simulink model "final_model_test"  (R2015a)
settings: Solver=ode3  StartTime=0.0  StopTime=10  RelTol=1e-3
settings Model: Creator=BML  LastModifiedBy=BML
settings SolverCC: AutoInsertRateTranBlk=on
settings DebuggingCC: AlgebraicLoopMsg=error  ArtificialAlgebraicLoopMsg=none  MaxConsecutiveZCsMsg=none
settings ModelReferenceCC: ModelReferenceMinAlgLoopOccurrences=on

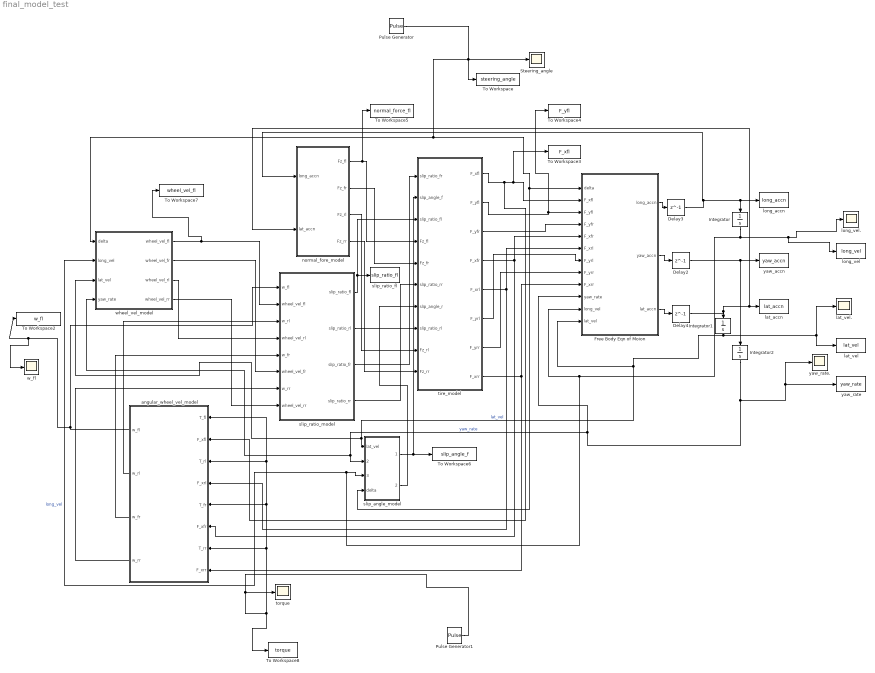
== system final_model_test ==
  "           Steering_angle" : Scope
      settings: SaveName=ScopeData8
  "           torque" : Scope
      settings: SaveName=ScopeData10
  Delay2 : Delay  DelayLength=1  SampleTime=1
  Delay3 : Delay  DelayLength=1  SampleTime=1
  Delay4 : Delay  DelayLength=1  SampleTime=1
  Free Body Eqn of Moion : Subsystem
  Integrator : Integrator  InitialCondition=22.22
  Integrator1 : Integrator
  Integrator2 : Integrator
  Pulse Generator : DiscretePulseGenerator  PulseType=Time based  Amplitude=0  Period=8  PulseWidth=5  PhaseDelay=3
  Pulse Generator1 : DiscretePulseGenerator  Amplitude=50  Period=8  PulseWidth=5  PhaseDelay=3
  To Workspace : ToWorkspace  VariableName=steering_angle  SaveFormat=Timeseries  SampleTime=1
  To Workspace2 : ToWorkspace  VariableName=w_fl  SaveFormat=Timeseries  SampleTime=1
  To Workspace3 : ToWorkspace  VariableName=F_xfl  SaveFormat=Timeseries  SampleTime=1
  To Workspace4 : ToWorkspace  VariableName=F_yfl  SaveFormat=Timeseries  SampleTime=1
  To Workspace5 : ToWorkspace  VariableName=normal_force_fl  SaveFormat=Timeseries  SampleTime=1
  To Workspace6 : ToWorkspace  VariableName=slip_angle_f  SaveFormat=Timeseries  SampleTime=1
  To Workspace7 : ToWorkspace  VariableName=wheel_vel_fl  SaveFormat=Timeseries  SampleTime=1
  To Workspace8 : ToWorkspace  VariableName=torque  SaveFormat=Timeseries  SampleTime=-1
  angular_wheel_vel_model : Subsystem
  lat_accn : ToWorkspace  VariableName=lat_accn  SaveFormat=Timeseries  SampleTime=1
  lat_vel : ToWorkspace  VariableName=lat_vel  SaveFormat=Timeseries  SampleTime=1
  lat_vel. : Scope
  long_accn : ToWorkspace  VariableName=long_accn  SaveFormat=Timeseries  SampleTime=1
  long_vel : ToWorkspace  VariableName=long_vel  SaveFormat=Timeseries  SampleTime=1
  long_vel. : Scope
  normal_fore_model : Subsystem
  slip_angle_model : Subsystem
  slip_ratio_fl : ToWorkspace  VariableName=slip_ratio_fl  SaveFormat=Timeseries  SampleTime=1
  slip_ratio_model : Subsystem
  tire_model : Subsystem
  w_fl : Scope
      settings: SaveName=ScopeData5
  wheel_vel_model : Subsystem
  yaw_accn : ToWorkspace  VariableName=yaw_accn  SaveFormat=Timeseries  SampleTime=1
  yaw_rate : ToWorkspace  VariableName=yaw_rate  SaveFormat=Timeseries  SampleTime=1
  yaw_rate. : Scope
      settings: SaveName=ScopeData2
  wires:
  slip_ratio_model/1(slip_ratio_fl) -> slip_ratio_fl/1, tire_model/3(slip_ratio_fl)
  slip_ratio_model/2(slip_ratio_rl) -> tire_model/8(slip_ratio_rl)
  Integrator2/1 -> Free Body Eqn of Moion/10(yaw_rate), slip_angle_model/2(yaw_rate), wheel_vel_model/4(yaw_rate), yaw_rate./1, yaw_rate/1  "yaw_rate"
  normal_fore_model/1(Fz_fl) -> To Workspace5/1, tire_model/4(Fz_fl)
  normal_fore_model/2(Fz_fr) -> tire_model/5(Fz_fr)
  normal_fore_model/3(Fz_rl) -> tire_model/9(Fz_rl)
  normal_fore_model/4(Fz_rr) -> tire_model/10(Fz_rr)
  wheel_vel_model/3(wheel_vel_rl) -> slip_ratio_model/4(wheel_vel_rl)
  slip_ratio_model/3(slip_ratio_fr) -> tire_model/1(slip_ratio_fr)
  slip_ratio_model/4(slip_ratio_rr) -> tire_model/6(slip_ratio_rr)
  slip_angle_model/1(slip_angle_f) -> To Workspace6/1, tire_model/2("slip_angle_f  ")
  slip_angle_model/2(slip_angle_r) -> tire_model/7(slip_angle_r)
  wheel_vel_model/2(wheel_vel_fr) -> slip_ratio_model/6(wheel_vel_fr)
  wheel_vel_model/1(wheel_vel_fl) -> To Workspace7/1, slip_ratio_model/2(wheel_vel_fl)
  wheel_vel_model/4(wheel_vel_rr) -> slip_ratio_model/8(wheel_vel_rr)
  Pulse Generator/1 -> "           Steering_angle"/1, To Workspace/1, slip_angle_model/4(delta), Free Body Eqn of Moion/1(delta), wheel_vel_model/1(delta)
  Integrator/1 -> Free Body Eqn of Moion/11(long_vel), slip_angle_model/3(long_vel), wheel_vel_model/2(long_vel), long_vel/1, long_vel./1  "long_vel"
  Integrator1/1 -> Free Body Eqn of Moion/12(lat_vel), wheel_vel_model/3(lat_vel), slip_angle_model/1(lat_vel), lat_vel./1, lat_vel/1  "lat_vel"
  Pulse Generator1/1 -> angular_wheel_vel_model/7(T_rr), angular_wheel_vel_model/5(T_fr), angular_wheel_vel_model/3(T_rl), angular_wheel_vel_model/1(T_fl), To Workspace8/1, "           torque"/1
  Free Body Eqn of Moion/2(yaw_accn) -> Delay2/1
  Free Body Eqn of Moion/1(long_accn) -> Delay3/1
  Free Body Eqn of Moion/3(lat_accn) -> Delay4/1
  angular_wheel_vel_model/4(w_rr) -> slip_ratio_model/7(w_rr)
  tire_model/3(F_yfr) -> Free Body Eqn of Moion/4(F_yfr)
  tire_model/6(F_yrl) -> Free Body Eqn of Moion/7(F_yrl)
  tire_model/7(F_yrr) -> Free Body Eqn of Moion/8(F_yrr)
  tire_model/2(F_yfl) -> To Workspace4/1, Free Body Eqn of Moion/3(F_yfl)
  Delay3/1 -> normal_fore_model/1(long_accn), Integrator/1, long_accn/1
  Delay4/1 -> normal_fore_model/2(lat_accn), lat_accn/1, Integrator1/1
  angular_wheel_vel_model/1(w_fl) -> slip_ratio_model/1(w_fl), w_fl/1, To Workspace2/1
  angular_wheel_vel_model/2(w_rl) -> slip_ratio_model/3(w_rl)
  angular_wheel_vel_model/3(w_fr) -> slip_ratio_model/5(w_fr)
  tire_model/1(F_xfl) -> angular_wheel_vel_model/2(F_xfl), To Workspace3/1, Free Body Eqn of Moion/2(F_xfl)
  tire_model/5(F_xrl) -> angular_wheel_vel_model/4(F_xrl), Free Body Eqn of Moion/6(F_xrl)
  tire_model/4(F_xfr) -> angular_wheel_vel_model/6(F_xfr), Free Body Eqn of Moion/5(F_xfr)
  tire_model/8(F_xrr) -> angular_wheel_vel_model/8(F_xrr), Free Body Eqn of Moion/9(F_xrr)
  Delay2/1 -> Integrator2/1, yaw_accn/1

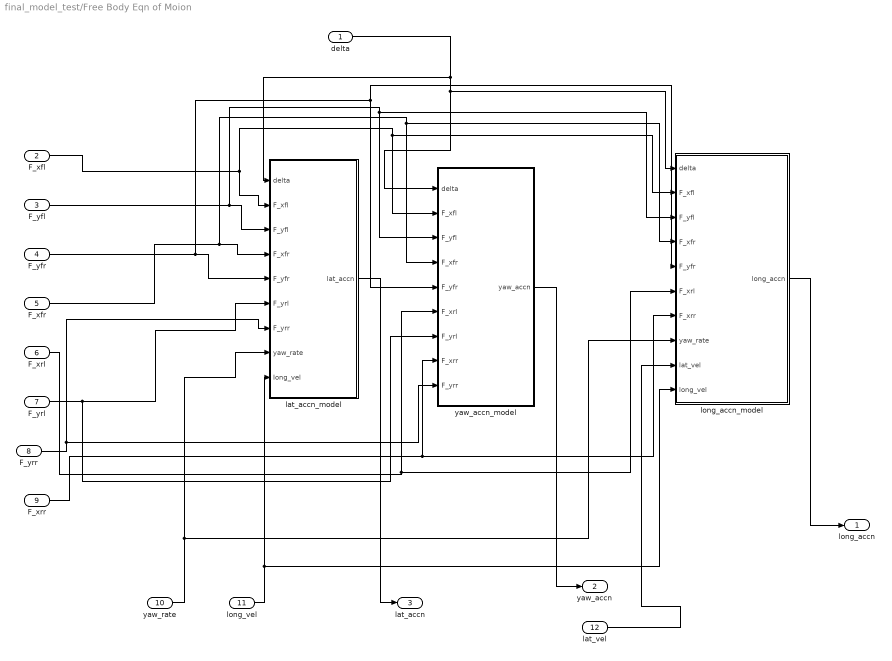
== system final_model_test/Free Body Eqn of Moion ==
  delta : Inport
  F_xfl : Inport  Port=2
  F_yfl : Inport  Port=3
  F_yfr : Inport  Port=4
  F_xfr : Inport  Port=5
  F_xrl : Inport  Port=6
  F_yrl : Inport  Port=7
  F_yrr : Inport  Port=8
  F_xrr : Inport  Port=9
  yaw_rate : Inport  Port=10
  long_vel : Inport  Port=11
  lat_vel : Inport  Port=12
  lat_accn_model : Subsystem
  long_accn_model : Subsystem
  yaw_accn_model : Subsystem
  long_accn : Outport
  yaw_accn : Outport  Port=2
  lat_accn : Outport  Port=3
  wires:
  yaw_rate/1 -> long_accn_model/8(yaw_rate), lat_accn_model/8(yaw_rate)
  long_vel/1 -> long_accn_model/10(long_vel), lat_accn_model/9(Iong_vel)
  lat_vel/1 -> long_accn_model/9(lat_vel)
  lat_accn_model/1(lat_accn) -> lat_accn/1
  F_yfl/1 -> long_accn_model/3(F_yfl), yaw_accn_model/3(F_yfl), lat_accn_model/3(F_yfl)
  delta/1 -> lat_accn_model/1(delta), yaw_accn_model/1(delta), long_accn_model/1(delta)
  F_xfr/1 -> long_accn_model/4(F_xfr), yaw_accn_model/4(F_xfr), lat_accn_model/4(F_xfr)
  F_yrl/1 -> yaw_accn_model/7(F_yrl), lat_accn_model/6(F_yrl)
  long_accn_model/1(long_accn) -> long_accn/1
  F_yfr/1 -> yaw_accn_model/5(F_yfr), long_accn_model/5(F_yfr), lat_accn_model/5(F_yfr)
  yaw_accn_model/1(yaw_accn) -> yaw_accn/1
  F_yrr/1 -> lat_accn_model/7(F_yrr), yaw_accn_model/9(F_yrr)
  F_xrl/1 -> long_accn_model/6(F_xrl), yaw_accn_model/6(F_xrl)
  F_xrr/1 -> long_accn_model/7(F_xrr), yaw_accn_model/8(F_xrr)
  F_xfl/1 -> long_accn_model/2(F_xfl), yaw_accn_model/2(F_xfl), lat_accn_model/2(F_xfl)

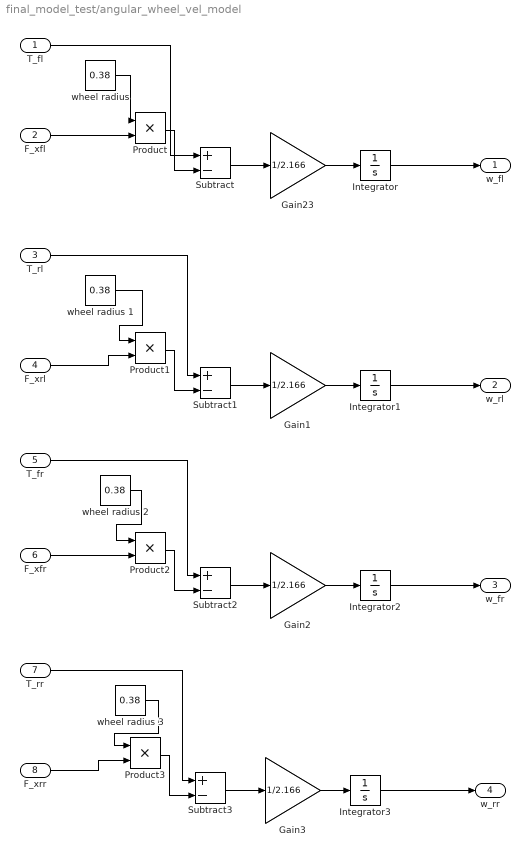
== system final_model_test/angular_wheel_vel_model ==
  T_fl : Inport
  F_xfl : Inport  Port=2
  T_rl : Inport  Port=3
  F_xrl : Inport  Port=4
  T_fr : Inport  Port=5
  F_xfr : Inport  Port=6
  T_rr : Inport  Port=7
  F_xrr : Inport  Port=8
  Gain{1..3,23} (4 alike) : Gain  Gain=1/2.166
  Integrator : Integrator  InitialCondition=58.5  LimitOutput=on  LowerSaturationLimit=1
  Integrator1 : Integrator  InitialCondition=58.5  LimitOutput=on  LowerSaturationLimit=57
  Integrator2 : Integrator  InitialCondition=58.5  LimitOutput=on  LowerSaturationLimit=57
  Integrator3 : Integrator  InitialCondition=58.5  LimitOutput=on  LowerSaturationLimit=57
  Product{,1..3} (4 alike) : Product
  Subtract{,1..3} (4 alike) : Sum  Inputs=+-
  wheel radius {,1..3} (4 alike) : Constant  Value=0.38
  w_fl : Outport
  w_rl : Outport  Port=2
  w_fr : Outport  Port=3
  w_rr : Outport  Port=4
  wires:
  Gain23/1 -> Integrator/1
  F_xfl/1 -> Product/2
  Product/1 -> Subtract/2
  wheel radius 1/1 -> Product1/1
  T_rl/1 -> Subtract1/1
  T_fl/1 -> Subtract/1
  Subtract/1 -> Gain23/1
  F_xrl/1 -> Product1/2
  "wheel radius "/1 -> Product/1
  Subtract2/1 -> Gain2/1
  wheel radius 2/1 -> Product2/1
  Product1/1 -> Subtract1/2
  F_xrr/1 -> Product3/2
  T_rr/1 -> Subtract3/1
  Gain3/1 -> Integrator3/1
  Subtract1/1 -> Gain1/1
  Gain1/1 -> Integrator1/1
  Gain2/1 -> Integrator2/1
  Subtract3/1 -> Gain3/1
  wheel radius 3/1 -> Product3/1
  F_xfr/1 -> Product2/2
  Product3/1 -> Subtract3/2
  T_fr/1 -> Subtract2/1
  Product2/1 -> Subtract2/2
  Integrator/1 -> w_fl/1
  Integrator1/1 -> w_rl/1
  Integrator2/1 -> w_fr/1
  Integrator3/1 -> w_rr/1

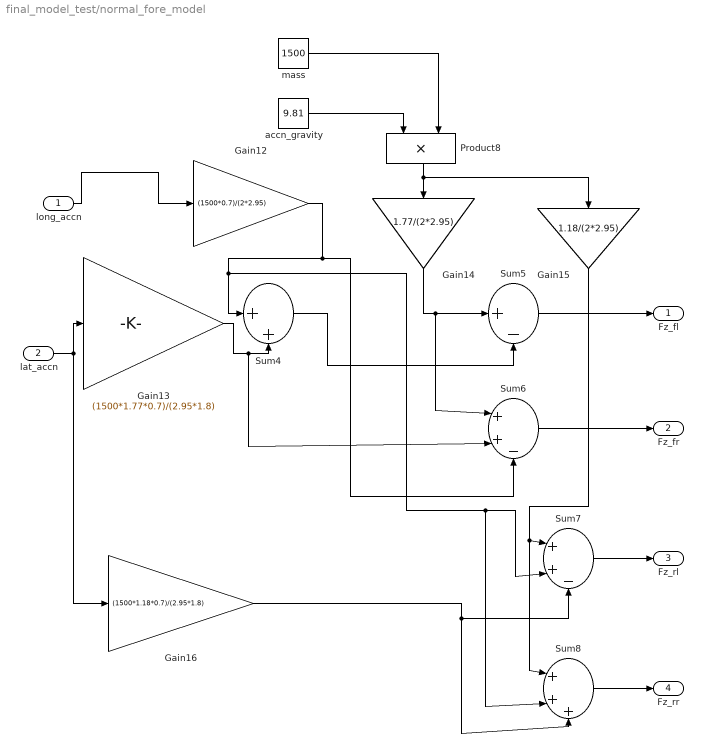
== system final_model_test/normal_fore_model ==
  long_accn : Inport
  lat_accn : Inport  Port=2
  Gain12 : Gain  Gain=(1500*0.7)/(2*2.95)
  Gain13 : Gain  Gain=(1500*1.77*0.7)/(2.95*1.8)
  Gain14 : Gain  Gain=1.77/(2*2.95)
  Gain15 : Gain  Gain=1.18/(2*2.95)
  Gain16 : Gain  Gain=(1500*1.18*0.7)/(2.95*1.8)
  Product8 : Product
  Sum4 : Sum  Inputs=|++
  Sum5 : Sum  Inputs=|+-
  Sum6 : Sum  Inputs=|++-
  Sum7 : Sum  Inputs=|++-
  Sum8 : Sum  Inputs=|+++
  "accn_gravity " : Constant  Value=9.81
  mass : Constant  Value=1500
  Fz_fl : Outport
  Fz_fr : Outport  Port=2
  Fz_rl : Outport  Port=3
  Fz_rr : Outport  Port=4
  wires:
  Gain12/1 -> Sum4/1, Sum8/2, Sum7/2, Sum6/3
  Gain15/1 -> Sum8/1, Sum7/1
  Gain16/1 -> Sum8/3, Sum7/3
  Sum7/1 -> Fz_rl/1
  lat_accn/1 -> Gain13/1, Gain16/1
  Gain13/1 -> Sum6/2, Sum4/2
  Sum5/1 -> Fz_fl/1
  Sum6/1 -> Fz_fr/1
  Sum4/1 -> Sum5/2
  long_accn/1 -> Gain12/1
  mass/1 -> Product8/2
  Gain14/1 -> Sum5/1, Sum6/1
  Sum8/1 -> Fz_rr/1
  Product8/1 -> Gain14/1, Gain15/1
  "accn_gravity "/1 -> Product8/1

== system final_model_test/slip_angle_model ==
  lat_vel : Inport
  yaw_rate : Inport  Port=2
  long_vel : Inport  Port=3
  delta : Inport  Port=4
  Divide4 : Product  Inputs=*/
  Divide5 : Product  Inputs=*/
  Product : Product
  Product1 : Product
  Sum4 : Sum  Inputs=|++
  Sum5 : Sum  Inputs=|+-
  Sum6 : Sum  Inputs=|+-
  l_f : Constant  Value=1.18
  l_r : Constant  Value=1.77
  slip_angle_f : Outport
  slip_angle_r : Outport  Port=2
  wires:
  yaw_rate/1 -> Product1/2, Product/2
  long_vel/1 -> Divide5/2, Divide4/2
  l_f/1 -> Product/1
  lat_vel/1 -> Sum6/2, Sum4/1
  Divide4/1 -> Sum5/2
  Product/1 -> Sum4/2
  Sum4/1 -> Divide4/1
  Divide5/1 -> slip_angle_r/1
  delta/1 -> Sum5/1
  Sum5/1 -> slip_angle_f/1
  Product1/1 -> Sum6/1
  l_r/1 -> Product1/1
  Sum6/1 -> Divide5/1

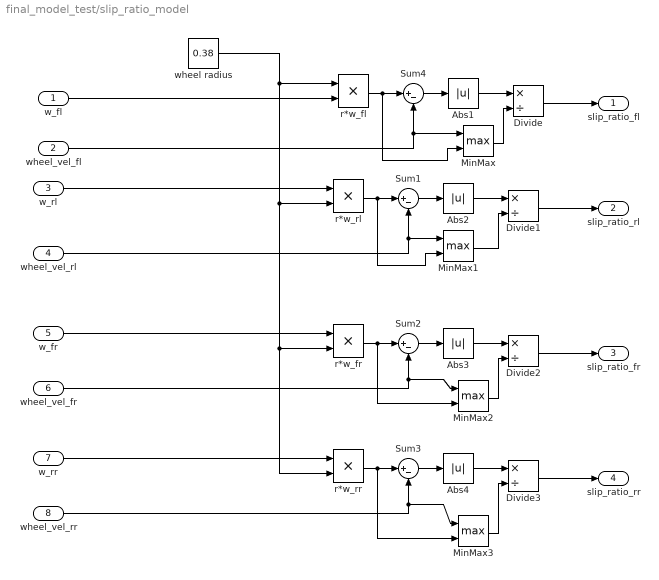
== system final_model_test/slip_ratio_model ==
  w_fl : Inport
  wheel_vel_fl : Inport  Port=2
  w_rl : Inport  Port=3
  wheel_vel_rl : Inport  Port=4
  w_fr : Inport  Port=5
  wheel_vel_fr : Inport  Port=6
  w_rr : Inport  Port=7
  wheel_vel_rr : Inport  Port=8
  Abs{1..4} (4 alike) : Abs
  Divide{,1..3} (4 alike) : Product  Inputs=*/
  MinMax{,1..3} (4 alike) : MinMax  Function=max  Inputs=2
  Sum{1..4} (4 alike) : Sum  Inputs=|+-
  r*w_fl : Product  Inputs=**
  r*w_fr : Product  Inputs=**
  r*w_rl : Product  Inputs=**
  r*w_rr : Product  Inputs=**
  wheel radius : Constant  Value=0.38
  slip_ratio_fl : Outport
  slip_ratio_rl : Outport  Port=2
  slip_ratio_fr : Outport  Port=3
  slip_ratio_rr : Outport  Port=4
  wires:
  w_fl/1 -> r*w_fl/2
  r*w_fl/1 -> MinMax/2, Sum4/1
  wheel radius/1 -> r*w_fl/1, r*w_rl/2, r*w_rr/2, r*w_fr/2
  wheel_vel_fl/1 -> Sum4/2, MinMax/1
  Sum4/1 -> Abs1/1
  Abs1/1 -> Divide/1
  MinMax/1 -> Divide/2
  Divide/1 -> slip_ratio_fl/1
  r*w_rl/1 -> MinMax1/2, Sum1/1
  wheel_vel_rl/1 -> Sum1/2, MinMax1/1
  Sum1/1 -> Abs2/1
  Abs2/1 -> Divide1/1
  MinMax1/1 -> Divide1/2
  Divide1/1 -> slip_ratio_rl/1
  w_rl/1 -> r*w_rl/1
  r*w_fr/1 -> MinMax2/2, Sum2/1
  wheel_vel_fr/1 -> MinMax2/1, Sum2/2
  Sum2/1 -> Abs3/1
  Abs3/1 -> Divide2/1
  MinMax2/1 -> Divide2/2
  Divide2/1 -> slip_ratio_fr/1
  w_fr/1 -> r*w_fr/1
  r*w_rr/1 -> MinMax3/2, Sum3/1
  wheel_vel_rr/1 -> MinMax3/1, Sum3/2
  Sum3/1 -> Abs4/1
  Abs4/1 -> Divide3/1
  MinMax3/1 -> Divide3/2
  Divide3/1 -> slip_ratio_rr/1
  w_rr/1 -> r*w_rr/1

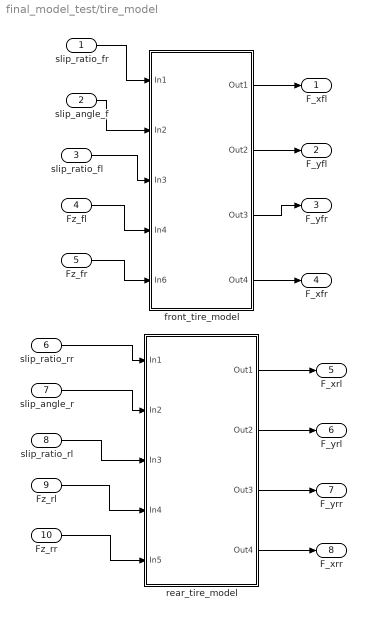
== system final_model_test/tire_model ==
  slip_ratio_fr : Inport
  "slip_angle_f  " : Inport  Port=2
  slip_ratio_fl : Inport  Port=3
  Fz_fl : Inport  Port=4
  Fz_fr : Inport  Port=5
  slip_ratio_rr : Inport  Port=6
  slip_angle_r : Inport  Port=7
  slip_ratio_rl : Inport  Port=8
  Fz_rl : Inport  Port=9
  Fz_rr : Inport  Port=10
  front_tire_model : Subsystem
  rear_tire_model : Subsystem
  F_xfl : Outport
  F_yfl : Outport  Port=2
  F_yfr : Outport  Port=3
  F_xfr : Outport  Port=4
  F_xrl : Outport  Port=5
  F_yrl : Outport  Port=6
  F_yrr : Outport  Port=7
  F_xrr : Outport  Port=8
  wires:
  slip_ratio_rr/1 -> rear_tire_model/1(In1)
  slip_angle_r/1 -> rear_tire_model/2(In2)
  rear_tire_model/3(Out3) -> F_yrr/1
  slip_ratio_rl/1 -> rear_tire_model/3(In3)
  rear_tire_model/2(Out2) -> F_yrl/1
  Fz_rr/1 -> rear_tire_model/5(In5)
  rear_tire_model/1(Out1) -> F_xrl/1
  rear_tire_model/4(Out4) -> F_xrr/1
  Fz_rl/1 -> rear_tire_model/4(In4)
  "slip_angle_f  "/1 -> front_tire_model/2(In2)
  slip_ratio_fr/1 -> front_tire_model/1(In1)
  slip_ratio_fl/1 -> front_tire_model/3(In3)
  Fz_fr/1 -> front_tire_model/5(In6)
  front_tire_model/1(Out1) -> F_xfl/1
  front_tire_model/3(Out3) -> F_yfr/1
  front_tire_model/2(Out2) -> F_yfl/1
  Fz_fl/1 -> front_tire_model/4(In4)
  front_tire_model/4(Out4) -> F_xfr/1

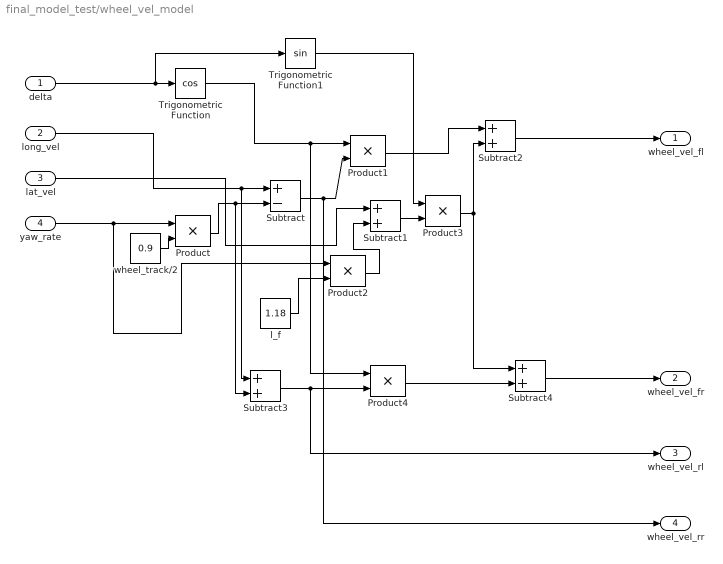
== system final_model_test/wheel_vel_model ==
  delta : Inport
  long_vel : Inport  Port=2
  lat_vel : Inport  Port=3
  yaw_rate : Inport  Port=4
  Product{,1..4} (5 alike) : Product
  Subtract : Sum  Inputs=+-
  Subtract{1..4} (4 alike) : Sum
  Trigonometric Function : Trigonometry  Operator=cos
  Trigonometric Function1 : Trigonometry
  l_f : Constant  Value=1.18
  wheel_track/2 : Constant  Value=0.9
  wheel_vel_fl : Outport
  wheel_vel_fr : Outport  Port=2
  wheel_vel_rl : Outport  Port=3
  wheel_vel_rr : Outport  Port=4
  wires:
  long_vel/1 -> Subtract3/1, Subtract/1
  l_f/1 -> Product2/2
  Subtract3/1 -> wheel_vel_rl/1, Product4/2
  Trigonometric Function/1 -> Product4/1, Product1/1
  Subtract1/1 -> Product3/2
  Subtract/1 -> wheel_vel_rr/1, Product1/2
  Product4/1 -> Subtract4/2
  Subtract4/1 -> wheel_vel_fr/1
  lat_vel/1 -> Subtract1/1
  Product/1 -> Subtract3/2, Subtract/2
  Product2/1 -> Subtract1/2
  Product1/1 -> Subtract2/1
  yaw_rate/1 -> Product/1, Product2/1
  wheel_track/2/1 -> Product/2
  Trigonometric Function1/1 -> Product3/1
  Subtract2/1 -> wheel_vel_fl/1
  delta/1 -> Trigonometric Function1/1, Trigonometric Function/1
  Product3/1 -> Subtract2/2, Subtract4/1

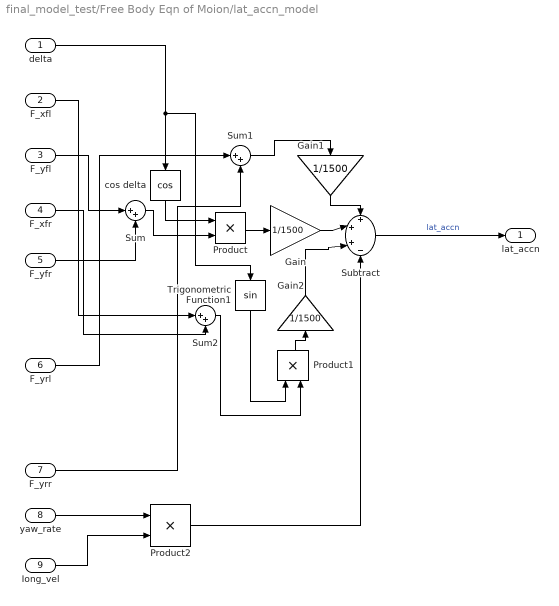
== system final_model_test/Free Body Eqn of Moion/lat_accn_model ==
  delta : Inport
  F_xfl : Inport  Port=2
  F_yfl : Inport  Port=3
  F_xfr : Inport  Port=4
  F_yfr : Inport  Port=5
  F_yrl : Inport  Port=6
  F_yrr : Inport  Port=7
  yaw_rate : Inport  Port=8
  Iong_vel : Inport  Port=9
  Gain : Gain  Gain=1/1500
  Gain1 : Gain  Gain=1/1500
  Gain2 : Gain  Gain=1/1500
  Product : Product
  Product1 : Product
  Product2 : Product
  Subtract : Sum  Inputs=+++-
  Sum : Sum  Inputs=|++
  Sum1 : Sum  Inputs=|++
  Sum2 : Sum  Inputs=|++
  Trigonometric Function1 : Trigonometry
  cos delta : Trigonometry  Operator=cos
  lat_accn : Outport
  wires:
  Gain/1 -> Subtract/2
  cos delta/1 -> Product/1
  Sum/1 -> Product/2
  Gain1/1 -> Subtract/1
  Sum1/1 -> Gain1/1
  Product/1 -> Gain/1
  delta/1 -> Trigonometric Function1/1, cos delta/1
  Trigonometric Function1/1 -> Product1/1
  Sum2/1 -> Product1/2
  Subtract/1 -> lat_accn/1  "lat_accn"
  Product2/1 -> Subtract/4
  Product1/1 -> Gain2/1
  F_xfr/1 -> Sum2/2
  F_xfl/1 -> Sum2/1
  Gain2/1 -> Subtract/3
  F_yfr/1 -> Sum/2
  F_yrl/1 -> Sum1/1
  yaw_rate/1 -> Product2/1
  F_yfl/1 -> Sum/1
  F_yrr/1 -> Sum1/2
  Iong_vel/1 -> Product2/2

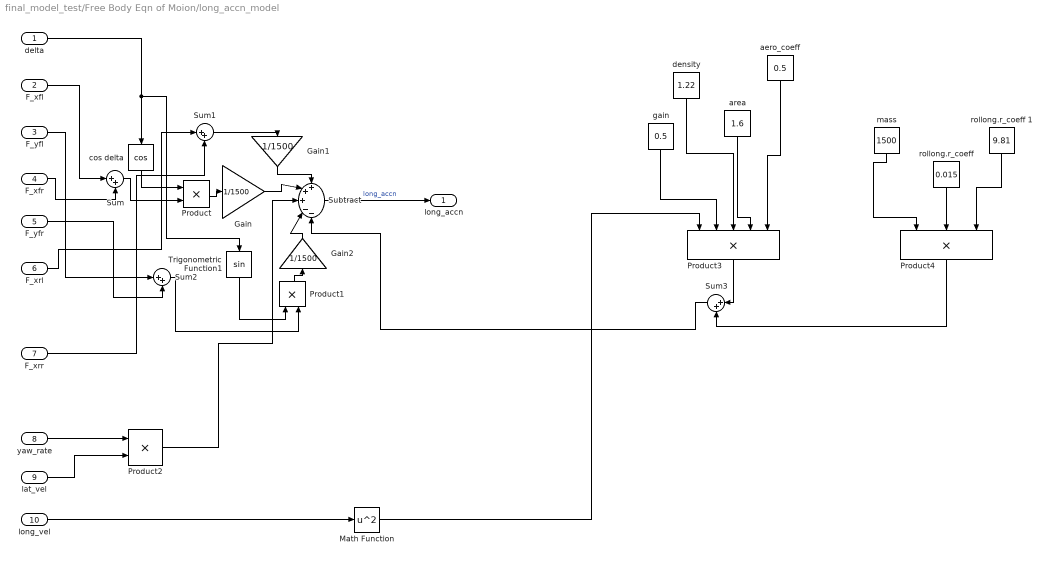
== system final_model_test/Free Body Eqn of Moion/long_accn_model ==
  delta : Inport
  F_xfl : Inport  Port=2
  F_yfl : Inport  Port=3
  F_xfr : Inport  Port=4
  F_yfr : Inport  Port=5
  F_xrl : Inport  Port=6
  F_xrr : Inport  Port=7
  yaw_rate : Inport  Port=8
  lat_vel : Inport  Port=9
  long_vel : Inport  Port=10
  Gain : Gain  Gain=1/1500
  Gain1 : Gain  Gain=1/1500
  Gain2 : Gain  Gain=1/1500
  Math Function : Math  Operator=square  SaturateOnIntegerOverflow=on
  Product : Product
  Product1 : Product
  Product2 : Product
  Product3 : Product  Inputs=5
  Product4 : Product  Inputs=3
  Subtract : Sum  Inputs=+++--
  Sum{,1..3} (4 alike) : Sum  Inputs=|++
  Trigonometric Function1 : Trigonometry
  "aero_coeff " : Constant  Value=0.5
  "area " : Constant  Value=1.6
  cos delta : Trigonometry  Operator=cos
  "density " : Constant  Value=1.22
  gain : Constant  Value=0.5
  mass : Constant  Value=1500
  "rollong.r_coeff " : Constant  Value=0.015
  rollong.r_coeff 1 : Constant  Value=9.81
  long_accn : Outport
  wires:
  Product2/1 -> Subtract/3
  Gain/1 -> Subtract/2
  cos delta/1 -> Product/1
  Sum/1 -> Product/2
  Product/1 -> Gain/1
  Gain1/1 -> Subtract/1
  F_xrr/1 -> Sum1/2
  Sum1/1 -> Gain1/1
  F_xfr/1 -> Sum/2
  F_xrl/1 -> Sum1/1
  F_xfl/1 -> Sum/1
  F_yfl/1 -> Sum2/1
  F_yfr/1 -> Sum2/2
  Product1/1 -> Gain2/1
  delta/1 -> Trigonometric Function1/1, cos delta/1
  Trigonometric Function1/1 -> Product1/1
  Subtract/1 -> long_accn/1  "long_accn"
  Sum2/1 -> Product1/2
  Gain2/1 -> Subtract/4
  yaw_rate/1 -> Product2/1
  lat_vel/1 -> Product2/2
  gain/1 -> Product3/2
  "density "/1 -> Product3/3
  "area "/1 -> Product3/4
  "aero_coeff "/1 -> Product3/5
  mass/1 -> Product4/1
  "rollong.r_coeff "/1 -> Product4/2
  rollong.r_coeff 1/1 -> Product4/3
  Math Function/1 -> Product3/1
  Product3/1 -> Sum3/1
  Product4/1 -> Sum3/2
  Sum3/1 -> Subtract/5
  long_vel/1 -> Math Function/1

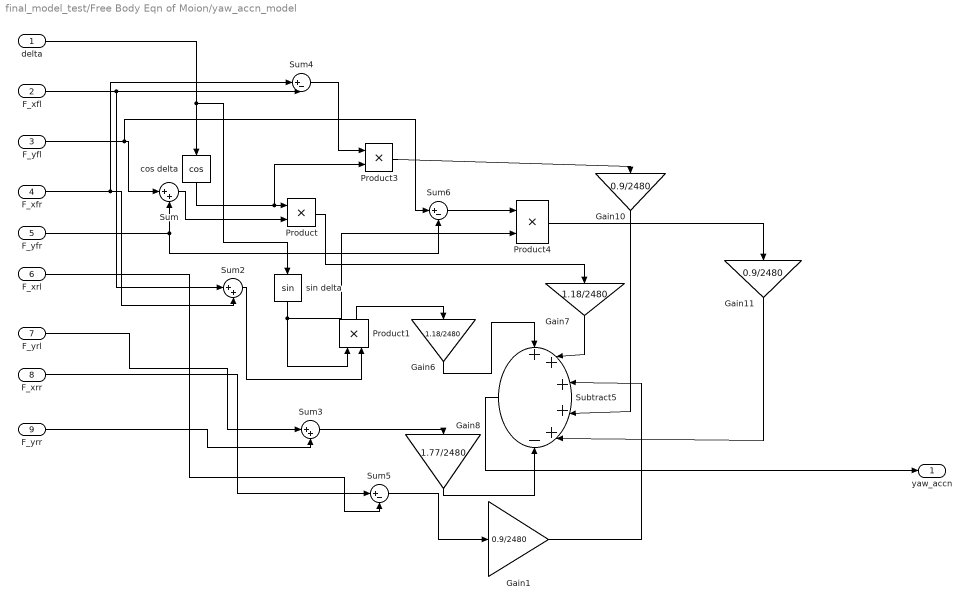
== system final_model_test/Free Body Eqn of Moion/yaw_accn_model ==
  delta : Inport
  F_xfl : Inport  Port=2
  F_yfl : Inport  Port=3
  F_xfr : Inport  Port=4
  F_yfr : Inport  Port=5
  F_xrl : Inport  Port=6
  F_yrl : Inport  Port=7
  F_xrr : Inport  Port=8
  F_yrr : Inport  Port=9
  Gain1 : Gain  Gain=0.9/2480
  Gain10 : Gain  Gain=0.9/2480
  Gain11 : Gain  Gain=0.9/2480
  Gain6 : Gain  Gain=1.18/2480
  Gain7 : Gain  Gain=1.18/2480
  Gain8 : Gain  Gain=1.77/2480
  Product{,1,3..4} (4 alike) : Product
  Subtract5 : Sum  Inputs=+++++-
  Sum : Sum  Inputs=|++
  Sum2 : Sum  Inputs=|++
  Sum3 : Sum  Inputs=|++
  Sum4 : Sum  Inputs=|+-
  Sum5 : Sum  Inputs=|+-
  Sum6 : Sum  Inputs=|+-
  cos delta : Trigonometry  Operator=cos
  "sin delta " : Trigonometry
  yaw_accn : Outport
  wires:
  Sum4/1 -> Product3/1
  delta/1 -> "sin delta "/1, cos delta/1
  F_yrl/1 -> Sum3/1
  Product3/1 -> Gain10/1
  Gain10/1 -> Subtract5/4
  F_xrr/1 -> Sum5/1
  F_yfl/1 -> Sum6/1, Sum/1
  Gain11/1 -> Subtract5/5
  F_yrr/1 -> Sum3/2
  F_xrl/1 -> Sum5/2
  "sin delta "/1 -> Product4/2, Product1/1
  cos delta/1 -> Product3/2, Product/1
  Gain7/1 -> Subtract5/2
  F_yfr/1 -> Sum6/2, Sum/2
  Gain6/1 -> Subtract5/1
  Gain8/1 -> Subtract5/6
  Product/1 -> Gain7/1
  F_xfl/1 -> Sum2/1, Sum4/2
  Product1/1 -> Gain6/1
  Sum3/1 -> Gain8/1
  Sum/1 -> Product/2
  Sum2/1 -> Product1/2
  F_xfr/1 -> Sum4/1, Sum2/2
  Sum6/1 -> Product4/1
  Subtract5/1 -> yaw_accn/1
  Sum5/1 -> Gain1/1
  Gain1/1 -> Subtract5/3
  Product4/1 -> Gain11/1

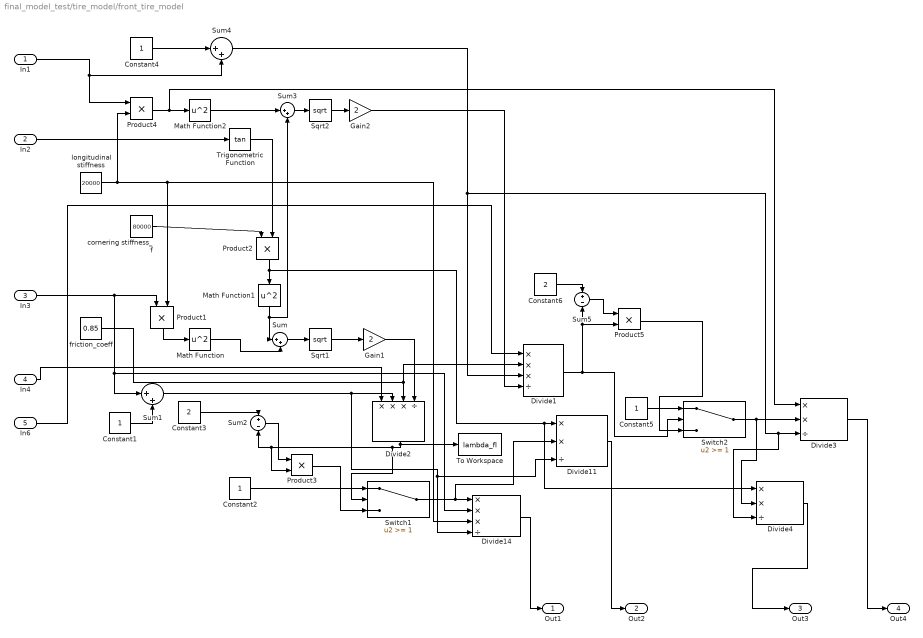
== system final_model_test/tire_model/front_tire_model ==
  In1 : Inport
  In2 : Inport  Port=2
  In3 : Inport  Port=3
  In4 : Inport  Port=4
  In6 : Inport  Port=5
  Constant{1..2,4..5} (4 alike) : Constant
  Constant3 : Constant  Value=2
  Constant6 : Constant  Value=2
  Divide1 : Product  Inputs=***/
  Divide11 : Product  Inputs=**/
  Divide14 : Product  Inputs=***/
  Divide2 : Product  Inputs=***/
  Divide3 : Product  Inputs=**/
  Divide4 : Product  Inputs=**/
  Gain1 : Gain  Gain=2
  Gain2 : Gain  Gain=2
  Math Function : Math  Operator=square  SaturateOnIntegerOverflow=on
  Math Function1 : Math  Operator=square  SaturateOnIntegerOverflow=on
  Math Function2 : Math  Operator=square  SaturateOnIntegerOverflow=on
  Product{1..5} (5 alike) : Product
  Sqrt1 : Sqrt  SaturateOnIntegerOverflow=on
  Sqrt2 : Sqrt  SaturateOnIntegerOverflow=on
  Sum{,1,3..4} (4 alike) : Sum  Inputs=|++
  Sum2 : Sum  Inputs=+-
  Sum5 : Sum  Inputs=+-
  Switch1 : Switch  Threshold=1
  Switch2 : Switch  Threshold=1
  To Workspace : ToWorkspace  VariableName=lambda_fl  SaveFormat=Timeseries  SampleTime=-1
  Trigonometric Function : Trigonometry  Operator=tan
  cornering stiffness_f : Constant  Value=80000
  friction_coeff : Constant  Value=0.85
  longitudinal stiffness : Constant  Value=20000
  Out1 : Outport
  Out2 : Outport  Port=2
  Out3 : Outport  Port=3
  Out4 : Outport  Port=4
  wires:
  Math Function/1 -> Sum/2
  Constant1/1 -> Sum1/2
  Gain1/1 -> Divide2/4
  Trigonometric Function/1 -> Product2/2
  In3/1 -> Divide14/2, Sum1/1, Product1/1
  Sum/1 -> Sqrt1/1
  friction_coeff/1 -> Divide1/2, Divide2/3
  Sqrt1/1 -> Gain1/1
  In4/1 -> Divide2/1
  Product3/1 -> Switch1/3
  Gain2/1 -> Divide1/4
  Math Function1/1 -> Sum3/2, Sum/1
  Sum5/1 -> Product5/1
  Product2/1 -> Divide4/1, Divide11/1, Math Function1/1
  Constant5/1 -> Switch2/1
  cornering stiffness_f/1 -> Product2/1
  Switch2/1 -> Divide4/2, Divide3/2
  In6/1 -> Divide1/1
  Sum4/1 -> Divide4/3, Divide3/3, Divide1/3
  Constant2/1 -> Switch1/1
  Sum1/1 -> Divide11/3, Divide14/4, Divide2/2
  In1/1 -> Sum4/2, Product4/1
  Switch1/1 -> Divide11/2, Divide14/1
  Constant4/1 -> Sum4/1
  longitudinal stiffness/1 -> Product4/2, Product1/2, Divide14/3
  Sum3/1 -> Sqrt2/1
  Math Function2/1 -> Sum3/1
  Constant6/1 -> Sum5/1
  Sqrt2/1 -> Gain2/1
  Product4/1 -> Divide3/1, Math Function2/1
  Sum2/1 -> Product3/1
  Divide1/1 -> Switch2/2, Sum5/2, Product5/2
  Constant3/1 -> Sum2/1
  Product1/1 -> Math Function/1
  In2/1 -> Trigonometric Function/1
  Divide2/1 -> Switch1/2, Product3/2, Sum2/2, To Workspace/1
  Product5/1 -> Switch2/3
  Divide14/1 -> Out1/1
  Divide3/1 -> Out4/1
  Divide11/1 -> Out2/1
  Divide4/1 -> Out3/1

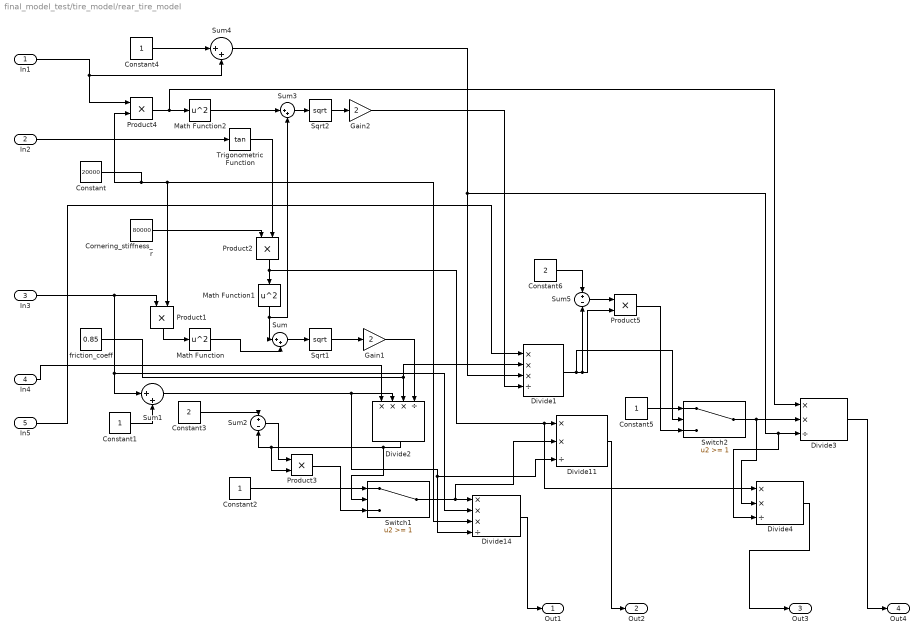
== system final_model_test/tire_model/rear_tire_model ==
  In1 : Inport
  In2 : Inport  Port=2
  In3 : Inport  Port=3
  In4 : Inport  Port=4
  In5 : Inport  Port=5
  Constant : Constant  Value=20000
  Constant{1..2,4..5} (4 alike) : Constant
  Constant3 : Constant  Value=2
  Constant6 : Constant  Value=2
  "Cornering_stiffness_r          " : Constant  Value=80000
  Divide1 : Product  Inputs=***/
  Divide11 : Product  Inputs=**/
  Divide14 : Product  Inputs=***/
  Divide2 : Product  Inputs=***/
  Divide3 : Product  Inputs=**/
  Divide4 : Product  Inputs=**/
  Gain1 : Gain  Gain=2
  Gain2 : Gain  Gain=2
  Math Function : Math  Operator=square  SaturateOnIntegerOverflow=on
  Math Function1 : Math  Operator=square  SaturateOnIntegerOverflow=on
  Math Function2 : Math  Operator=square  SaturateOnIntegerOverflow=on
  Product{1..5} (5 alike) : Product
  Sqrt1 : Sqrt  SaturateOnIntegerOverflow=on
  Sqrt2 : Sqrt  SaturateOnIntegerOverflow=on
  Sum{,1,3..4} (4 alike) : Sum  Inputs=|++
  Sum2 : Sum  Inputs=+-
  Sum5 : Sum  Inputs=+-
  Switch1 : Switch  Threshold=1
  Switch2 : Switch  Threshold=1
  Trigonometric Function : Trigonometry  Operator=tan
  friction_coeff : Constant  Value=0.85
  Out1 : Outport
  Out2 : Outport  Port=2
  Out3 : Outport  Port=3
  Out4 : Outport  Port=4
  wires:
  Sum2/1 -> Product3/1
  In4/1 -> Divide2/1
  Divide2/1 -> Switch1/2, Product3/2, Sum2/2
  Product3/1 -> Switch1/3
  Constant3/1 -> Sum2/1
  Constant2/1 -> Switch1/1
  friction_coeff/1 -> Divide1/2, Divide2/3
  Sum1/1 -> Divide11/3, Divide14/4, Divide2/2
  Constant/1 -> Product4/2, Product1/2, Divide14/3
  Gain1/1 -> Divide2/4
  Constant4/1 -> Sum4/1
  Product2/1 -> Divide4/1, Divide11/1, Math Function1/1
  Sum3/1 -> Sqrt2/1
  Sqrt2/1 -> Gain2/1
  Gain2/1 -> Divide1/4
  In1/1 -> Sum4/2, Product4/1
  Math Function2/1 -> Sum3/1
  Sum5/1 -> Product5/1
  In5/1 -> Divide1/1
  Math Function1/1 -> Sum3/2, Sum/1
  "Cornering_stiffness_r          "/1 -> Product2/1
  Switch1/1 -> Divide11/2, Divide14/1
  Divide1/1 -> Switch2/2, Sum5/2, Product5/2
  Constant6/1 -> Sum5/1
  In3/1 -> Divide14/2, Sum1/1, Product1/1
  Product1/1 -> Math Function/1
  Trigonometric Function/1 -> Product2/2
  Sum/1 -> Sqrt1/1
  Sqrt1/1 -> Gain1/1
  Constant1/1 -> Sum1/2
  In2/1 -> Trigonometric Function/1
  Math Function/1 -> Sum/2
  Constant5/1 -> Switch2/1
  Product4/1 -> Divide3/1, Math Function2/1
  Product5/1 -> Switch2/3
  Switch2/1 -> Divide4/2, Divide3/2
  Sum4/1 -> Divide4/3, Divide3/3, Divide1/3
  Divide14/1 -> Out1/1
  Divide3/1 -> Out4/1
  Divide11/1 -> Out2/1
  Divide4/1 -> Out3/1
